simulink model "oke_Qudus_2"  (R2023b)
settings: Solver=VariableStepAuto  StartTime=0.0  StopTime=10.0  RelTol=1e-3
values from neighbouring files (symbols this model uses):
  Bt = 0.0869    [dc_machine_control_1.m]
  Hc = 0.355    [dc_machine_control_1.m]
  J = 0.0607    [dc_machine_control_1.m]
  Kb = 1.26    [dc_machine_control_1.m]
  Kc = 2.33    [dc_machine_control_1.m]
  Ks = 28.73    [dc_machine_control_1.m]
  Kw = 0.065    [dc_machine_control_1.m]
  La = 0.072    [dc_machine_control_1.m]
  Ra = 4    [dc_machine_control_1.m]
  Tc = 0.0208    [dc_machine_control_1.m]
  Ts = 0.0188    [dc_machine_control_1.m]
  Tw = 0.002    [dc_machine_control_1.m]
undefined symbols (not defined in the file or in its folder): D1, lagging, pulse
libraries: spsSeriesRLCBranchLib x3, spsACVoltageSourceLib x3, spsPLL3phLib x1, spsPulseGeneratorThyristor12PulseLib x1, spsUniversalBridgeLib x1, spsThreePhaseVIMeasurementLib x1, spsVoltageMeasurementLib x1, spsGroundLib x1, sps_lib x1
settings Model: Creator=USER  LastModifiedBy=USER

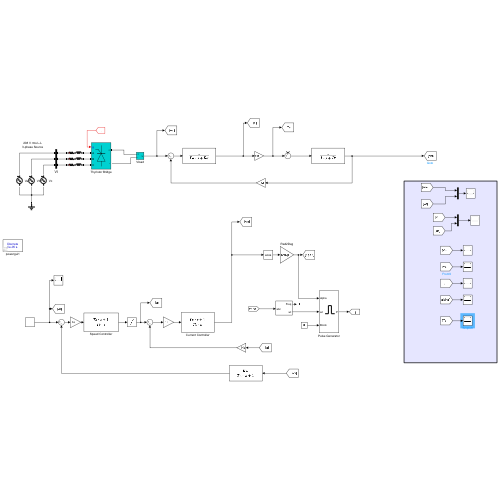
[thumbnail: Simulink's stored preview of the top-level diagram]
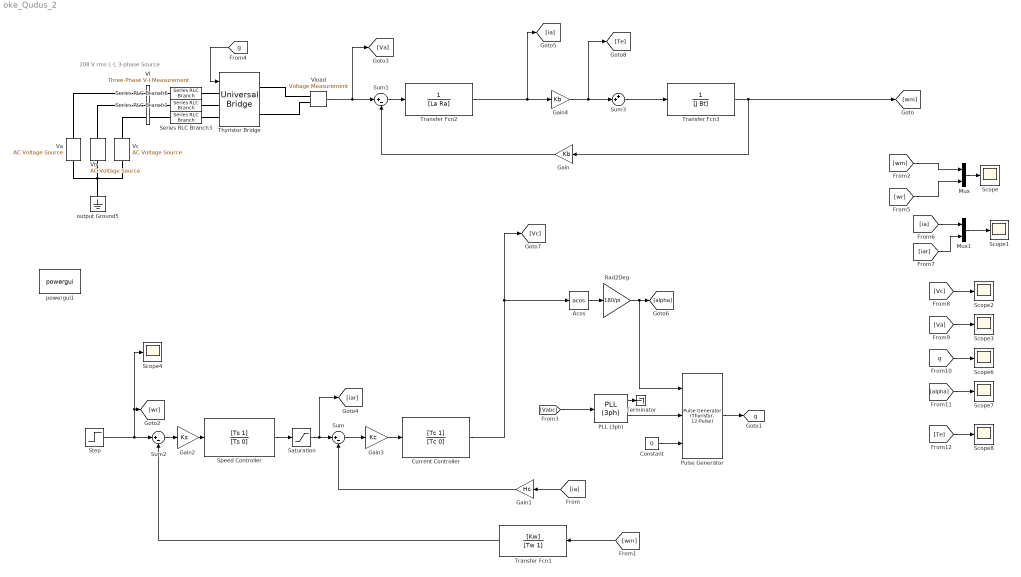
== system oke_Qudus_2 ==
  note: 208 V rms L-L
      | 3-phase Source
  Acos : Trigonometry  Operator=acos
  Constant : Constant  Value=0
  Current Controller : TransferFcn  Numerator=[Tc 1]  Denominator=[Tc 0]
  Gain : Gain  Gain=Kb
  Gain1 : Gain  Gain=Hc
  Gain2 : Gain  Gain=Ks
  Gain3 : Gain  Gain=Kc
  Gain4 : Gain  Gain=Kb
  Mux : Mux  Inputs=2
  Mux1 : Mux  Inputs=2
  PLL (3ph) : spsPLL3phLib/PLL (3ph)  Fmin=45  Par_Init=[0, 60]  ParK=[180, 3200, 1]  TcD=1e-4  MaxRateChangeFreq=12  FilterCutOffFreq=25  Ts=0  AGC=on
  Pulse Generator : spsPulseGeneratorThyristor12PulseLib/Pulse Generator (Thyristor, 12-Pulse)  GenType=6-pulse  Delta=D1 (lagging)  pwidth=10  Double_Pulse=on  Ts=0
      settings: LibrarySourceBlock=|
      | sps_lib/Power Electronics/Power Electronics Control/Pulse Generator
      | (Thyristor, 12-Pulse)
  Rad2Deg : Gain  Gain=180/pi  SaturateOnIntegerOverflow=on  OutDataTypeStr=Inherit: Same as input  ParamDataTypeStr=Inherit: Same as input
  Saturation : Saturate  UpperLimit=20  LowerLimit=0
  Scope{,1..4,6..8} (8 alike) : Scope
  Series RLC Branch1 : spsSeriesRLCBranchLib/Series RLC Branch  LConnTagsString=__new0  RConnTagsString=__new0  BranchType=RL  Resistance=0.01  Inductance=1e-3  SetiL0=off  InitialCurrent=0  Capacitance=[]  Setx0=off  InitialVoltage=0  Measurements=None
  Series RLC Branch3 : spsSeriesRLCBranchLib/Series RLC Branch  LConnTagsString=__new0  RConnTagsString=__new0  BranchType=RL  Resistance=0.01  Inductance=1e-3  SetiL0=off  InitialCurrent=0  Capacitance=[]  Setx0=off  InitialVoltage=0  Measurements=None
  Series RLC Branch6 : spsSeriesRLCBranchLib/Series RLC Branch  LConnTagsString=__new0  RConnTagsString=__new0  BranchType=RL  Resistance=0.01  Inductance=1e-3  SetiL0=off  InitialCurrent=0  Capacitance=[]  Setx0=off  InitialVoltage=0  Measurements=None
  Speed Controller : TransferFcn  Numerator=[Ts 1]  Denominator=[Ts 0]
  Step : Step  SampleTime=0
  Sum : Sum  Inputs=|+-
  Sum1 : Sum  Inputs=|+-
  Sum2 : Sum  Inputs=|+-
  Sum3 : Sum  Inputs=++|
  Terminator : Terminator
  Thyristor Bridge : spsUniversalBridgeLib/Universal Bridge  Arms=3  SnubberResistance=1e6  SnubberCapacitance=inf  Device=Thyristors  Ron=1e-3  Lon=0  ForwardVoltages="[  0  0  ]"  ForwardVoltage=0  GTOparameters=[ 10e-6 , 20e-6 ]  IGBTparameters=[ 1e-6 , 2e-6 ]  Measurements=None  Measurements_2=None  converterType=Rectifier
  Transfer Fcn1 : TransferFcn  Numerator=[Kw]  Denominator=[Tw 1]
  Transfer Fcn2 : TransferFcn  Denominator=[La Ra]
  Transfer Fcn3 : TransferFcn  Denominator=[J Bt]
  VI : spsThreePhaseVIMeasurementLib/Three-Phase V-I Measurement  VoltageMeasurement=phase-to-ground  SetLabelV=on  LabelV=Vabc  Vpu=on  VpuLL=off  CurrentMeasurement=yes  SetLabelI=on  LabelI=Iabc  Ipu=off  Pbase=100e6  Vbase=208  OutputType=Complex  PhasorSimulation=off  PSBequivalent=0
  Va : spsACVoltageSourceLib/AC Voltage Source  Description=source block  Amplitude=220  Phase=0  Frequency=60  SampleTime=0  Measurements=None  BusType=swing  Pref=10e3  Qref=0  Qmin=-inf  Qmax=+inf
      settings: AttributesFormatString=\n
  Vb : spsACVoltageSourceLib/AC Voltage Source  Description=source block  Amplitude=220  Phase=-120  Frequency=60  SampleTime=0  Measurements=None  BusType=swing  Pref=10e3  Qref=0  Qmin=-inf  Qmax=+inf
      settings: AttributesFormatString=\n
  Vc : spsACVoltageSourceLib/AC Voltage Source  Description=source block  Amplitude=220  Phase=120  Frequency=60  SampleTime=0  Measurements=None  BusType=swing  Pref=10e3  Qref=0  Qmin=-inf  Qmax=+inf
      settings: AttributesFormatString=\n
  Vload : spsVoltageMeasurementLib/Voltage Measurement  PhasorSimulation=off  OutputType=Complex  PSBequivalent=0
  output Ground5 : spsGroundLib/Ground  LConnTagsString=a
  powergui1 : sps_lib/powergui  Priority=1  SimulationMode=Discrete  SampleTime=50e-6  frequency=60  Iterations=50  frequencyindice=0  Pbase=100e6  ErrMax=1e-4  UnitsV=kV  UnitsW=MW  buscounter=0  FunctionMessages=off  echomessages=off  EnableUseOfTLC=off  CurrentSourceSwitches=off  DisableSnubberDevices=off  DisableRonSwitches=off  DisableVfSwitches=off  DisplayEquations=off  AutomaticDiscreteSolvers=off  SolverType=Tustin/Backward Euler (TBE)  Interpol=off  ExternalGateDelay=off  methode=off  Ts=10  x0status=blocks  SPID=off  SwTol=0  HookPort=off  NonlinearTolerance=1e-4  nMaxIteration=100  ContinueOnMaxIteration=off  RestoreLinks=warning  ResistiveCurrentMeasurement=off  Frange=[0:2:500]  Ylog=off  Xlog=on  ShowGrid=off  save=off  variable=ZData  structure=0  ZoomFFT=off  StartTime=0.0  cycles=1  DisplayStyle=1  fundamental=60  FreqAxis=off  MaxFrequency=1000  frequencyindicesteady=1  RmsSteady=1  display=off
  tag scope: g=global
  wires:
  Constant/1 -> Pulse Generator/3
  [g] -> Thyristor Bridge/1
  Pulse Generator/1 -> [g]
  [Vabc] -> PLL (3ph)/1
  PLL (3ph)/2 -> Pulse Generator/2
  PLL (3ph)/1 -> Terminator/1
  Saturation/1 -> [iar], Sum/1
  Step/1 -> Scope4/1, [wr], Sum2/1
  Speed Controller/1 -> Saturation/1
  Sum2/1 -> Gain2/1
  Gain3/1 -> Current Controller/1
  Transfer Fcn1/1 -> Sum2/2
  Gain2/1 -> Speed Controller/1
  Gain1/1 -> Sum/2
  Sum/1 -> Gain3/1
  Gain4/1 -> [Te], Sum3/2
  Gain/1 -> Sum1/2
  Transfer Fcn2/1 -> [ia], Gain4/1
  Vload/1 -> [Va], Sum1/1
  Sum3/1 -> Transfer Fcn3/1
  Sum1/1 -> Transfer Fcn2/1
  Transfer Fcn3/1 -> [wm], Gain/1
  [ia] -> Gain1/1
  [wm] -> Transfer Fcn1/1
  [Va] -> Scope3/1
  Mux1/1 -> Scope1/1
  [iar] -> Mux1/2
  [ia] -> Mux1/1
  [Vc] -> Scope2/1
  [wr] -> Mux/2
  [wm] -> Mux/1
  Mux/1 -> Scope/1
  Current Controller/1 -> [Vc], Acos/1
  Acos/1 -> Rad2Deg/1
  Rad2Deg/1 -> Pulse Generator/1, [alpha]
  [g] -> Scope6/1
  [alpha] -> Scope7/1
  [Te] -> Scope8/1
  connections:
  Vb/LConn1 -- output Ground5/LConn1 -- Vc/LConn1 -- Va/LConn1
  Va/RConn1 -- VI/LConn1
  VI/RConn2 -- Series RLC Branch1/LConn1
  Vc/RConn1 -- VI/LConn3
  VI/RConn3 -- Series RLC Branch3/LConn1
  VI/RConn1 -- Series RLC Branch6/LConn1
  Series RLC Branch6/RConn1 -- Thyristor Bridge/LConn1
  Series RLC Branch3/RConn1 -- Thyristor Bridge/LConn3
  Series RLC Branch1/RConn1 -- Thyristor Bridge/LConn2
  Vb/RConn1 -- VI/LConn2
  Vload/LConn1 -- Thyristor Bridge/RConn1
  Thyristor Bridge/RConn2 -- Vload/LConn2
